simulink model "CascadaBun"  (R2016a)
settings: Solver=VariableStepAuto  StartTime=0.0  StopTime=400  RelTol=1e-3
undefined symbols (not defined in the file): k, k1, k2, k3, keta
libraries: simulink x2
settings Model: Creator=Nico Jula  LastModifiedBy=Nico Jula

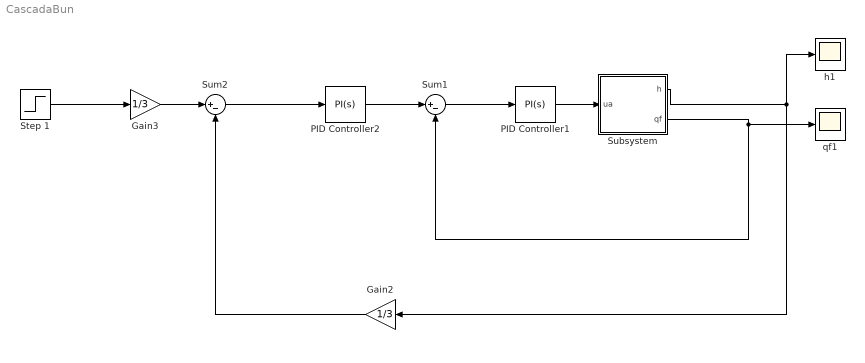
== system CascadaBun ==
  Gain2 : Gain  Gain=1/3
  Gain3 : Gain  Gain=1/3
  PID Controller1 : simulink/Continuous/PID Controller  Controller=PI  TimeDomain=Continuous-time  SampleTime=-1  IntegratorMethod=Forward Euler  FilterMethod=Forward Euler  Form=Parallel  UseFilter=on  ControllerParametersSource=internal  P=0.07  I=1  D=0  N=100  InitialConditionSource=internal  InitialConditionForIntegrator=5  InitialConditionForFilter=0  ExternalReset=none  LimitOutput=off  UpperSaturationLimit=inf  LowerSaturationLimit=-inf  LinearizeAsGain=on  AntiWindupMode=none  Kb=1  TrackingMode=off  Kt=1  PParamMin=[]  PParamMax=[]  IParamMin=[]  IParamMax=[]  DParamMin=[]  DParamMax=[]  NParamMin=[]  NParamMax=[]  KbParamMin=[]  KbParamMax=[]  KtParamMin=[]  KtParamMax=[]  POutMin=[]  POutMax=[]  IOutMin=[]  IOutMax=[]  DOutMin=[]  DOutMax=[]  NOutMin=[]  NOutMax=[]  KbOutMin=[]  KbOutMax=[]  KtOutMin=[]  KtOutMax=[]  IntegratorOutMin=[]  IntegratorOutMax=[]  FilterOutMin=[]  FilterOutMax=[]  SumOutMin=[]  SumOutMax=[]  SumI1OutMin=[]  SumI1OutMax=[]  SumI2OutMin=[]  SumI2OutMax=[]  SumI3OutMin=[]  SumI3OutMax=[]  SumDOutMin=[]  SumDOutMax=[]  SaturationOutMin=[]  SaturationOutMax=[]  IntegratorContinuousStateAttributes=''  IntegratorStateMustResolveToSignalObject=off  IntegratorRTWStateStorageClass=Auto  FilterContinuousStateAttributes=''  FilterStateMustResolveToSignalObject=off  FilterRTWStateStorageClass=Auto  DifferentiatorICPrevScaledInput=0  DifferentiatorOutMin=[]  DifferentiatorOutMax=[]
  PID Controller2 : simulink/Continuous/PID Controller  Controller=PI  TimeDomain=Continuous-time  SampleTime=-1  IntegratorMethod=Forward Euler  FilterMethod=Forward Euler  Form=Parallel  UseFilter=on  ControllerParametersSource=internal  P=40  I=0.16  D=0  N=100  InitialConditionSource=internal  InitialConditionForIntegrator=30  InitialConditionForFilter=0  ExternalReset=none  LimitOutput=off  UpperSaturationLimit=inf  LowerSaturationLimit=-inf  LinearizeAsGain=on  AntiWindupMode=none  Kb=1  TrackingMode=off  Kt=1  PParamMin=[]  PParamMax=[]  IParamMin=[]  IParamMax=[]  DParamMin=[]  DParamMax=[]  NParamMin=[]  NParamMax=[]  KbParamMin=[]  KbParamMax=[]  KtParamMin=[]  KtParamMax=[]  POutMin=[]  POutMax=[]  IOutMin=[]  IOutMax=[]  DOutMin=[]  DOutMax=[]  NOutMin=[]  NOutMax=[]  KbOutMin=[]  KbOutMax=[]  KtOutMin=[]  KtOutMax=[]  IntegratorOutMin=[]  IntegratorOutMax=[]  FilterOutMin=[]  FilterOutMax=[]  SumOutMin=[]  SumOutMax=[]  SumI1OutMin=[]  SumI1OutMax=[]  SumI2OutMin=[]  SumI2OutMax=[]  SumI3OutMin=[]  SumI3OutMax=[]  SumDOutMin=[]  SumDOutMax=[]  SaturationOutMin=[]  SaturationOutMax=[]  IntegratorContinuousStateAttributes=''  IntegratorStateMustResolveToSignalObject=off  IntegratorRTWStateStorageClass=Auto  FilterContinuousStateAttributes=''  FilterStateMustResolveToSignalObject=off  FilterRTWStateStorageClass=Auto  DifferentiatorICPrevScaledInput=0  DifferentiatorOutMin=[]  DifferentiatorOutMax=[]
  Step 1 : Step  Time=0  Before=10.8  After=13  SampleTime=0
  Subsystem : Subsystem
  Sum1 : Sum  Inputs=|+-
  Sum2 : Sum  Inputs=|+-
  h1 : Scope
  qf1 : Scope
  wires:
  PID Controller2/1 -> Sum1/1
  Sum1/1 -> PID Controller1/1
  Subsystem/1(h) -> h1/1, Gain2/1
  PID Controller1/1 -> Subsystem/1(ua)
  Subsystem/2(qf) -> Sum1/2, qf1/1
  Sum2/1 -> PID Controller2/1
  Gain2/1 -> Sum2/2
  Step 1/1 -> Gain3/1
  Gain3/1 -> Sum2/1

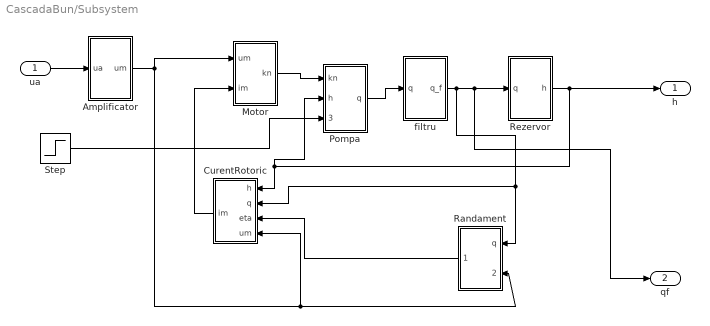
== system CascadaBun/Subsystem ==
  ua : Inport
  Amplificator : Subsystem
  CurentRotoric : Subsystem
  Motor : Subsystem
  Pompa : Subsystem
  Randament : Subsystem
  Rezervor : Subsystem
  Step : Step  Time=300  After=0.008  SampleTime=0
  filtru : Subsystem
  h : Outport
  qf : Outport  Port=2
  wires:
  Amplificator/1(um) -> CurentRotoric/4(um), Randament/2(um), Motor/1(um)
  CurentRotoric/1(im) -> Motor/2(im)
  Pompa/1(q) -> filtru/1(q)
  Rezervor/1(h) -> h/1, CurentRotoric/1(h), Pompa/2(h)
  filtru/1(q_f) -> qf/1, Rezervor/1(q), Randament/1(q), CurentRotoric/2(q)
  ua/1 -> Amplificator/1(ua)
  Randament/1(eta) -> CurentRotoric/3(eta)
  Motor/1("kn ") -> Pompa/1(kn)
  Step/1 -> Pompa/3("perturbatie k ")

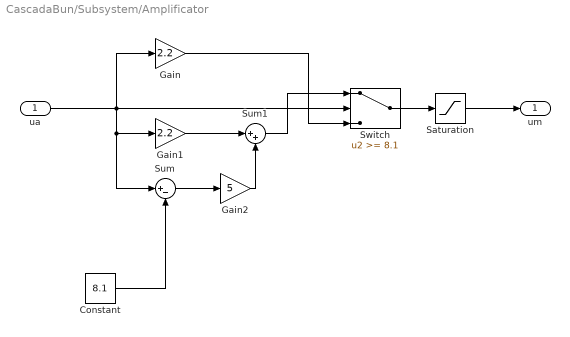
== system CascadaBun/Subsystem/Amplificator ==
  ua : Inport
  Constant : Constant  Value=8.1
  Gain : Gain  Gain=2.2
  Gain1 : Gain  Gain=2.2
  Gain2 : Gain  Gain=5
  Saturation : Saturate  UpperLimit=22  LowerLimit=0
  Sum : Sum  Inputs=|+-
  Sum1 : Sum  Inputs=|++
  Switch : Switch  Threshold=8.1
  um : Outport
  wires:
  Constant/1 -> Sum/2
  Saturation/1 -> um/1
  ua/1 -> Switch/2, Gain1/1, Sum/1, Gain/1
  Sum/1 -> Gain2/1
  Switch/1 -> Saturation/1
  Gain1/1 -> Sum1/1
  Sum1/1 -> Switch/1
  Gain/1 -> Switch/3
  Gain2/1 -> Sum1/2

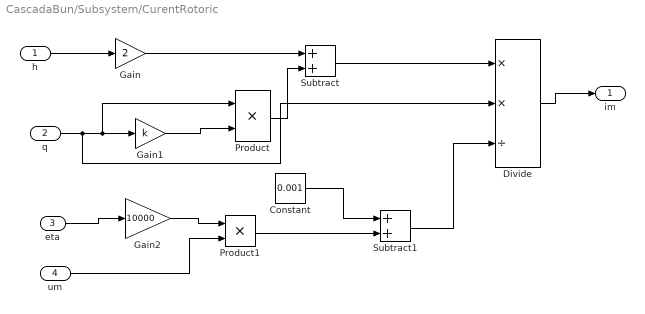
== system CascadaBun/Subsystem/CurentRotoric ==
  h : Inport
  q : Inport  Port=2
  eta : Inport  Port=3
  um : Inport  Port=4
  Constant : Constant  Value=0.001
  Divide : Product  Inputs=**/
  Gain : Gain  Gain=2
  Gain1 : Gain  Gain=k
  Gain2 : Gain  Gain=10000
  Product : Product
  Product1 : Product
  Subtract : Sum
  Subtract1 : Sum
  im : Outport
  wires:
  Gain2/1 -> Product1/1
  Subtract1/1 -> Divide/3
  Gain/1 -> Subtract/1
  q/1 -> Divide/2, Product/1, Gain1/1
  h/1 -> Gain/1
  Product/1 -> Subtract/2
  Constant/1 -> Subtract1/1
  Divide/1 -> im/1
  um/1 -> Product1/2
  Subtract/1 -> Divide/1
  Gain1/1 -> Product/2
  eta/1 -> Gain2/1
  Product1/1 -> Subtract1/2

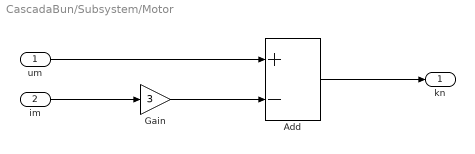
== system CascadaBun/Subsystem/Motor ==
  um : Inport
  im : Inport  Port=2
  Add : Sum  Inputs=+-
  Gain : Gain  Gain=3
  "kn " : Outport
  wires:
  im/1 -> Gain/1
  Add/1 -> "kn "/1
  Gain/1 -> Add/2
  um/1 -> Add/1

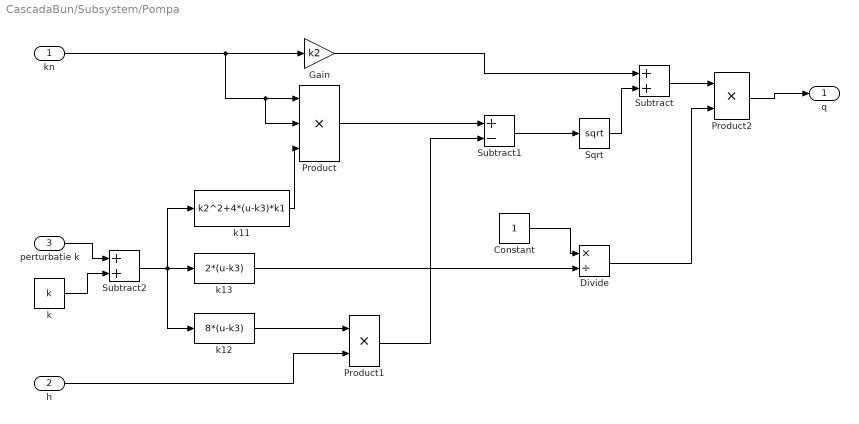
== system CascadaBun/Subsystem/Pompa ==
  kn : Inport
  h : Inport  Port=2
  "perturbatie k " : Inport  Port=3
  Constant : Constant
  Divide : Product  Inputs=*/
  Gain : Gain  Gain=k2
  Product : Product  Inputs=3
  Product1 : Product
  Product2 : Product
  Sqrt : Sqrt  SaturateOnIntegerOverflow=on
  Subtract : Sum
  Subtract1 : Sum  Inputs=+-
  Subtract2 : Sum
  k : Constant  Value=k
  k11 : Fcn  Expr=k2^2+4*(u-k3)*k1
  k12 : Fcn  Expr=8*(u-k3)
  k13 : Fcn  Expr=2*(u-k3)
  q : Outport
  wires:
  Subtract1/1 -> Sqrt/1
  Gain/1 -> Subtract/1
  Sqrt/1 -> Subtract/2
  kn/1 -> Product/1, Product/2, Gain/1
  "perturbatie k "/1 -> Subtract2/1
  k/1 -> Subtract2/2
  Subtract2/1 -> k12/1, k13/1, k11/1
  k11/1 -> Product/3
  k12/1 -> Product1/1
  h/1 -> Product1/2
  Product1/1 -> Subtract1/2
  Product/1 -> Subtract1/1
  Subtract/1 -> Product2/1
  Product2/1 -> q/1
  Constant/1 -> Divide/1
  k13/1 -> Divide/2
  Divide/1 -> Product2/2

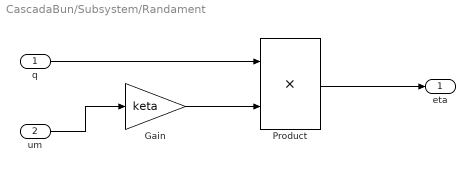
== system CascadaBun/Subsystem/Randament ==
  q : Inport
  um : Inport  Port=2
  Gain : Gain  Gain=keta
  Product : Product
  eta : Outport
  wires:
  um/1 -> Gain/1
  Product/1 -> eta/1
  Gain/1 -> Product/2
  q/1 -> Product/1

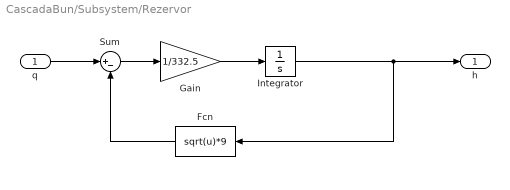
== system CascadaBun/Subsystem/Rezervor ==
  q : Inport
  Fcn : Fcn  Expr=sqrt(u)*9
  Gain : Gain  Gain=1/332.5
  Integrator : Integrator  InitialCondition=10.5
  Sum : Sum  Inputs=|+-
  h : Outport
  wires:
  Fcn/1 -> Sum/2
  Gain/1 -> Integrator/1
  Sum/1 -> Gain/1
  q/1 -> Sum/1
  Integrator/1 -> h/1, Fcn/1

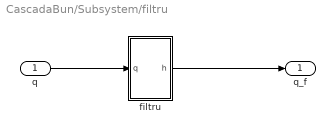
== system CascadaBun/Subsystem/filtru ==
  q : Inport
  filtru : Subsystem
  q_f : Outport
  wires:
  filtru/1(h) -> q_f/1
  q/1 -> filtru/1(q)

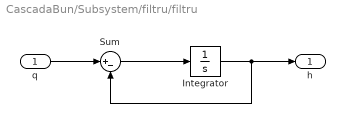
== system CascadaBun/Subsystem/filtru/filtru ==
  q : Inport
  Integrator : Integrator  InitialCondition=29.2
  Sum : Sum  Inputs=|+-
  h : Outport
  wires:
  Integrator/1 -> h/1, Sum/2
  q/1 -> Sum/1
  Sum/1 -> Integrator/1
